simulink library "calcThrTension_ul"  (R2020a)
settings: Solver=VariableStepAuto  StartTime=0.0  StopTime=10.0  RelTol=1e-3
libraries: simulink x1, vrlib x1, VectorMagnitude_ul x1
settings Model: Creator=Ayaz  LastModifiedBy=Ayaz

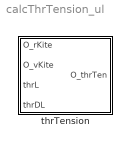
== system calcThrTension_ul ==
  thrTension : Subsystem  mask{thrSpringCns=10243}
      mask prompts: thrSpringCns "Tether spring constant [N/m]"

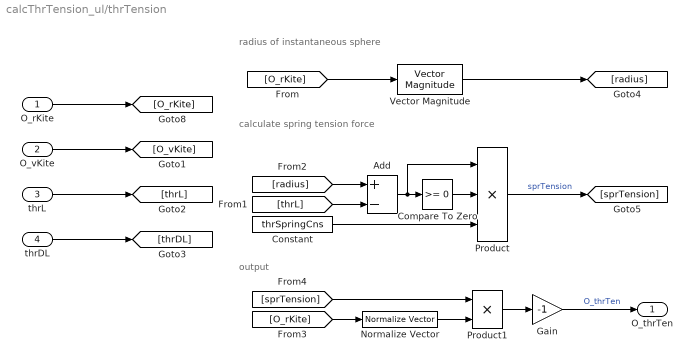
== system calcThrTension_ul/thrTension ==
  note: output
  note: calculate spring tension force
  note: radius of instantaneous sphere
  O_rKite : Inport
  O_vKite : Inport  Port=2
  thrL : Inport  Port=3
  thrDL : Inport  Port=4
  Add : Sum  Inputs=+-
  Compare To Zero : simulink/Logic and Bit Operations/Compare To Zero  relop=>=  OutDataTypeStr=boolean
  Constant : Constant  Value=thrSpringCns
  Gain : Gain  Gain=-1
  Normalize Vector : vrlib/Utilities/Normalize Vector  maxzero=0
  Product : Product  Inputs=3
  Product1 : Product
  Vector Magnitude : VectorMagnitude_ul/Vector Magnitude  SystemSampleTime=-1  Latency=0  AutoFrameSizeCalculation=off
  O_thrTen : Outport
  wires:
  O_rKite/1 -> [O_rKite]
  O_vKite/1 -> [O_vKite]
  thrL/1 -> [thrL]
  thrDL/1 -> [thrDL]
  Vector Magnitude/1 -> [radius]
  [radius] -> Add/1
  [thrL] -> Add/2
  Add/1 -> Product/1, Compare To Zero/1
  Compare To Zero/1 -> Product/2
  Product/1 -> [sprTension]  "sprTension"
  [O_rKite] -> Normalize Vector/1
  Normalize Vector/1 -> Product1/2
  [sprTension] -> Product1/1
  Product1/1 -> Gain/1
  Gain/1 -> O_thrTen/1  "O_thrTen"
  Constant/1 -> Product/3
  [O_rKite] -> Vector Magnitude/1
